simulink model "FGA1"  (R2015a)
settings: Solver=ode45  SolverMode=SingleTasking  StartTime=0.0  StopTime=10.0  RelTol=1e-3
undefined symbols (not defined in the file or in its folder): CW_ALgo
libraries: fuzblock x2
settings Model: CovSFcnEnable=off  Creator=Nauman  LastModifiedBy=Nauman
settings DataIOCC: SaveOutput=off  SaveTime=off
settings OptimizationCC: BlockReduction=off  BooleanDataType=off
settings DebuggingCC: SaveWithParameterizedLinksMsg=none  UnderspecifiedInitializationDetection=Classic  MergeDetectMultiDrivingBlocksExec=none  SignalResolutionControl=TryResolveAllWithWarning
settings HardwareCC: TargetUnknown=on

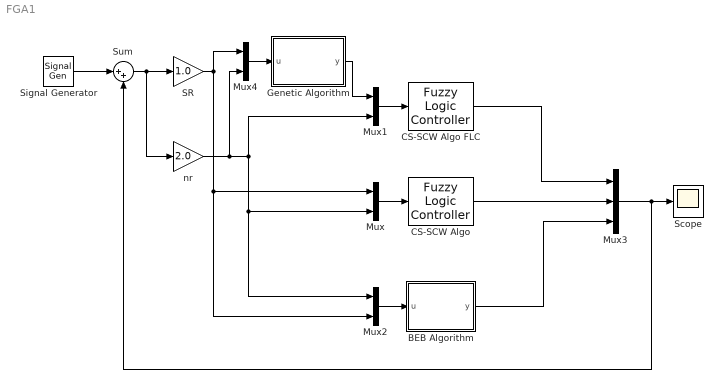
== system FGA1 ==
  BEB Algorithm : MATLAB Function  TreatAsAtomicUnit=on
  CS-SCW Algo : fuzblock/Fuzzy Logic  Controller  fis=[CW_ALgo.fis]
  CS-SCW Algo FLC : fuzblock/Fuzzy Logic  Controller  fis=[CW_ALgo.fis]
  Genetic Algorithm : MATLAB Function  TreatAsAtomicUnit=on
  Mux{,1..2,4} (4 alike) : Mux  Inputs=2
  Mux3 : Mux  Inputs=3
  SR : Gain  Gain=1.0  ParamMin=[0]  ParamMax=[1]  OutMin=[0]  OutMax=[1]
  Scope : Scope
  Signal Generator : SignalGenerator  WaveForm=random  Units=rad/sec  VectorParams1D=off
  Sum : Sum  Inputs=|++
  nr : Gain  Gain=2.0  ParamMin=[1]  ParamMax=[6]  OutMin=[1]  OutMax=[6]
  wires:
  SR/1 -> Mux2/2, Mux/1, Mux4/1
  Sum/1 -> nr/1, SR/1
  Signal Generator/1 -> Sum/1
  Genetic Algorithm/1(y) -> Mux1/1
  Mux1/1 -> CS-SCW Algo FLC/1
  Mux/1 -> CS-SCW Algo/1
  Mux2/1 -> BEB Algorithm/1(u)
  CS-SCW Algo FLC/1 -> Mux3/1
  BEB Algorithm/1(y) -> Mux3/3
  CS-SCW Algo/1 -> Mux3/2
  Mux3/1 -> Sum/2, Scope/1
  nr/1 -> Mux4/2, Mux1/2, Mux/2, Mux2/1
  Mux4/1 -> Genetic Algorithm/1(u)

== matlab function FGA1/BEB Algorithm ==
  data: u input; y output
function y = fcn(u)
%#codegen

y = u;

== matlab function FGA1/Genetic Algorithm ==
  data: u input; y output
function y = fcn(u)
%#codegen

y = u;
